simulink model "Planta_5_8_24"  (R2021a)
settings: Solver=VariableStepAuto  StartTime=0.0  StopTime=130  FixedStep=0.002  MaxStep=1e-3  RelTol=1e-4
model workspace (MAT data in the model file):
  VelMin = 0.5
  vMax = -0.3
values from neighbouring files (symbols this model uses):
  ax_max = 0.8    [valoresPlanta_29_9_24.m]    (also in valoresPlanta_v4.m)
  ay_max = 0.75    [valoresPlanta_29_9_24.m]    (also in valoresPlanta_v4.m)
  bcy = 1e7    (= 10000000)    [Valores_1.m]    (also in valoresPlanta.m; valoresPlanta_29_9_24.m; valoresPlanta_V3.m; valoresPlanta_v4.m)
  bh_eq = bhm*ih^2+bhd    (= 8720)    [Valores.m]    (also in Valores_1.m; valoresPlanta.m; valoresPlanta_29_9_24.m; valoresPlanta_V3.m)
  bhb = 1e8    (= 100000000)    [Valores.m]    (also in Valores_1.m; valoresPlanta.m; valoresPlanta_29_9_24.m; valoresPlanta_V3.m)
  bhEb = 2.2e9    (= 2200000000)    [Valores.m]    (also in Valores_1.m; valoresPlanta.m; valoresPlanta_29_9_24.m; valoresPlanta_V3.m)
  bt = 90.0    (= 90)    [Valores.m]    (also in Valores_1.m; valoresPlanta.m; valoresPlanta_29_9_24.m; valoresPlanta_V3.m)
  bt_eq = btd+(btm*(it^2))    (= 5401.8)    [valoresPlanta.m]    (also in valoresPlanta_29_9_24.m; valoresPlanta_V3.m; valoresPlanta_v4.m)
  btb = 5e6    (= 5000000)    [Valores.m]    (also in Valores_1.m; valoresPlanta.m; valoresPlanta_29_9_24.m; valoresPlanta_V3.m)
  btw = 3.0e3    (= 3000)    [Valores.m]    (also in Valores_1.m; valoresPlanta.m; valoresPlanta_29_9_24.m; valoresPlanta_V3.m)
  bwu = 150    [Valores.m]    (also in Valores_1.m; valoresPlanta.m; valoresPlanta_29_9_24.m; valoresPlanta_V3.m)
  estado_cont = [x_positions; hy_cont]    [perfilObsaculos.m]    (also in valoresPlanta_29_9_24.m = [x_positions; [hy_muelle hy_cont]]; valoresPlanta_v4.m = [x_positions; [hy_muelle hy_cont]])
  g = 9.80665    [Valores.m]    (also in Valores_1.m; valoresPlanta.m; valoresPlanta_29_9_24.m; valoresPlanta_V3.m)
  Hc = 0    [Valores.m]    (also in Valores_1.m = 2.5; valoresPlanta.m = 2.5; valoresPlanta_29_9_24.m = 2.5; valoresPlanta_V3.m = 2.5)
  hx_cont = 2.5    [perfilObsaculos.m]    (also in puntosTrayectoria.m; valoresPlanta_29_9_24.m; valoresPlanta_v4.m)
  ih = 22    [Valores.m]    (also in Valores_1.m; valoresPlanta.m; valoresPlanta_29_9_24.m; valoresPlanta_V3.m)
  it = 30    [Valores.m]    (also in Valores_1.m; valoresPlanta.m; valoresPlanta_29_9_24.m; valoresPlanta_V3.m)
  Jh_eq = Jhm_hb*ih^2+Jhd_hEb    (= 18320)    [Valores.m]    (also in Valores_1.m; valoresPlanta.m; valoresPlanta_29_9_24.m; valoresPlanta_V3.m)
  Jt_eq = Jtd+(Jtm_tb*(it^2))    (= 7500)    [valoresPlanta.m]    (also in valoresPlanta_29_9_24.m; valoresPlanta_V3.m; valoresPlanta_v4.m)
  kcy = 1.8e9    (= 1800000000)    [Valores_1.m]    (also in valoresPlanta.m; valoresPlanta_29_9_24.m; valoresPlanta_V3.m; valoresPlanta_v4.m)
  KDh = Jeq2 * w_posh^3    (= -12245.4404091)    [Valores.m]    (also in Valores_1.m = Jeq2 * w_posh; valoresPlanta.m = Jeq2 * w_posh; valoresPlanta_29_9_24.m = Jh_eq * n * w_posh; valoresPlanta_V3.m = Jeq2 * w_posh)
  KDt = Meq2 * w_post^3    (= -4728.86946035)    [Valores.m]    (also in Valores_1.m = Meq2 * w_post; valoresPlanta.m = Meq2 * w_post; valoresPlanta_29_9_24.m = 10127; valoresPlanta_V3.m = Meq2 * w_post)
  KIh = Jeq2 * w_posh^2    (= 2572.66592082)    [Valores.m]    (also in Valores_1.m = Jeq2 * w_posh^3; valoresPlanta.m = Jeq2 * w_posh^3; valoresPlanta_29_9_24.m = Jh_eq * w_posh^3; valoresPlanta_V3.m = Jeq2 * w_posh^3)
  KIt = Meq2 * w_post^2    (= 1307.690244)    [Valores.m]    (also in Valores_1.m = Meq2 * w_post^3; valoresPlanta.m = Meq2 * w_post^3; valoresPlanta_29_9_24.m = 6809.6; valoresPlanta_V3.m = Meq2 * w_post^3)
  KPh = Jeq2 * w_posh    (= -540.495867769)    [Valores.m]    (also in Valores_1.m = Jeq2 * w_posh^2; valoresPlanta.m = Jeq2 * w_posh^2; valoresPlanta_29_9_24.m = Jh_eq * n * w_posh^2; valoresPlanta_V3.m = Jeq2 * w_posh^2)
  KPt = Meq2 * w_post    (= -361.62)    [Valores.m]    (also in Valores_1.m = Meq2 * w_post^2; valoresPlanta.m = Meq2 * w_post^2; valoresPlanta_29_9_24.m = 14123; valoresPlanta_V3.m = Meq2 * w_post^2)
  Ktw = 4.8e5    (= 480000)    [Valores.m]    (also in Valores_1.m; valoresPlanta.m; valoresPlanta_29_9_24.m; valoresPlanta_V3.m)
  kwu = 2.36e8    (= 236000000)    [Valores.m]    (also in Valores_1.m; valoresPlanta.m; valoresPlanta_29_9_24.m; valoresPlanta_V3.m)
  Mc_max = 5e4    (= 50000)    [Valores.m]    (also in Valores_1.m; valoresPlanta.m; valoresPlanta_29_9_24.m; valoresPlanta_V3.m)
  Mc_min = 2e3    (= 2000)    [Valores.m]    (also in Valores_1.m; valoresPlanta.m; valoresPlanta_29_9_24.m; valoresPlanta_V3.m)
  Meq = Mt+(it^2*Jtm_tb+Jtd)/rtd^2    (= 60000)    [Valores.m]    (also in Valores_1.m; valoresPlanta_29_9_24.m; valoresPlanta_v4.m)
  Ms = 1.5e4    (= 15000)    [Valores.m]    (also in Valores_1.m; valoresPlanta.m; valoresPlanta_29_9_24.m; valoresPlanta_V3.m)
  Mt = 30000    [Valores.m]    (also in Valores_1.m; valoresPlanta.m; valoresPlanta_29_9_24.m; valoresPlanta_V3.m)
  pos = [p0; p1; p2; p3; p4; p5]    [calcularTrayectoria2_prueba.m]    (also in perfilObsaculos.m = puntosTrayectoria(4, 1.5, 20, [-20,0], estado_cont, hy_cont,; puntosTrayectoria.m; valoresPlanta_29_9_24.m = calcularTrayectoria2_prueba(vx_max, vhmax, ax_max, Hc, hx_co; valoresPlanta_v4.m = calcularTrayectoria2_prueba(vx_max, vhmax, ax_max, Hc, hx_co)
  rhd = 0.75    [Valores.m]    (also in Valores_1.m; valoresPlanta.m; valoresPlanta_29_9_24.m; valoresPlanta_V3.m)
  rtd = 0.5    [Valores.m]    (also in Valores_1.m; valoresPlanta.m; valoresPlanta_29_9_24.m; valoresPlanta_V3.m)
  tau_hm = 1e-3    (= 0.001)    [valoresPlanta.m]    (also in valoresPlanta_29_9_24.m; valoresPlanta_V3.m; valoresPlanta_v4.m)
  tau_tm = 1e-3    (= 0.001)    [Valores.m]    (also in Valores_1.m; valoresPlanta.m; valoresPlanta_29_9_24.m; valoresPlanta_V3.m)
  Thb_Max = 5e4    (= 50000)    [Valores.m]    (also in Valores_1.m; valoresPlanta.m; valoresPlanta_29_9_24.m; valoresPlanta_V3.m)
  ThEb_Max = 1.1e6    (= 1100000)    [Valores.m]    (also in Valores_1.m; valoresPlanta.m; valoresPlanta_29_9_24.m; valoresPlanta_V3.m)
  Thm_Max = 2e4    (= 20000)    [Valores.m]    (also in Valores_1.m; valoresPlanta.m; valoresPlanta_29_9_24.m; valoresPlanta_V3.m)
  Ttb_Max = 5e3    (= 5000)    [Valores.m]    (also in Valores_1.m; valoresPlanta.m; valoresPlanta_29_9_24.m; valoresPlanta_V3.m)
  Ttm_Max = 3e3    (= 3000)    [Valores.m]    (also in Valores_1.m; valoresPlanta.m; valoresPlanta_29_9_24.m = 4000; valoresPlanta_V3.m)
  vhmax = 3    [valoresPlanta_29_9_24.m]    (also in valoresPlanta_V3.m; valoresPlanta_v4.m)
  vx_max = 4    [valoresPlanta_29_9_24.m]    (also in valoresPlanta_v4.m)
  whmMax = P/Thm_Max    (= 47.8075)    [Valores_1.m]    (also in valoresPlanta.m; valoresPlanta_29_9_24.m = 176; valoresPlanta_V3.m; valoresPlanta_v4.m = 176)
  whmMin = 0.02    [valoresPlanta_29_9_24.m]    (also in valoresPlanta_v4.m = 0.2)
  wtmMax = (4/rtd)*it    (= 240)    [Valores_1.m]    (also in valoresPlanta.m; valoresPlanta_29_9_24.m; valoresPlanta_V3.m; valoresPlanta_v4.m)
  wtmMin = 0.02    [valoresPlanta_29_9_24.m]    (also in valoresPlanta_v4.m = 0.2)
  x_0 = -20    [valoresPlanta_29_9_24.m]    (also in valoresPlanta_v4.m)
  x_0_tamb = x_0/rtd    (= -40)    [valoresPlanta_29_9_24.m]    (also in valoresPlanta_v4.m)
  xLimMax = 49    [valoresPlanta_29_9_24.m]    (also in valoresPlanta_v4.m)
  xLimMaxSeguridad = 50    [valoresPlanta_29_9_24.m]    (also in valoresPlanta_v4.m)
  xLimMin = -29    [valoresPlanta_29_9_24.m]    (also in valoresPlanta_v4.m)
  xLimMinSeguridad = -30    [valoresPlanta_29_9_24.m]    (also in valoresPlanta_v4.m)
  y_0 = 2.5    [valoresPlanta_29_9_24.m]    (also in valoresPlanta_v4.m)
  y_0_izaje = 3*(2/rhd)    (= 8)    [valoresPlanta_29_9_24.m]    (also in valoresPlanta_v4.m)
  yLimMax = 44    [valoresPlanta_29_9_24.m]    (also in valoresPlanta_v4.m)
  yLimMaxSeguridad = 45    [valoresPlanta_29_9_24.m]    (also in valoresPlanta_v4.m)
  yLimMin = -19    [valoresPlanta_29_9_24.m]    (also in valoresPlanta_v4.m)
  yLimMinSeguridad = -20    [valoresPlanta_29_9_24.m]    (also in valoresPlanta_v4.m)
  Yt0 = 45    [Valores.m]    (also in Valores_1.m; valoresPlanta.m; valoresPlanta_29_9_24.m; valoresPlanta_V3.m)
undefined symbols (not defined in the file or in its folder): DiscIntNeverNeededParam
libraries: simulink x3, vrlib x1, simulink_extras x1, aerolibanimutils x1
(part 2 of 3)

== system Planta_5_8_24/Planta/Modulador de Torque ==
  note: Modulador de Torque
  Ttm_ : Inport
  whd : Inport  Port=2
  wtd : Inport  Port=3
  T_hm_0 : Inport  Port=4
  Thm_ : Inport  Port=5
  Gain : Gain  Gain=bh_eq
  Gain1 : Gain  Gain=bt_eq
  Modulador de Torque Carro : Subsystem
  Modulador de Torque Izaje : Subsystem
  Saturation6 : Saturate  UpperLimit=Ttm_Max  LowerLimit=-Ttm_Max
  Saturation7 : Saturate  UpperLimit=Thm_Max  LowerLimit=-Thm_Max
  Scope29 : Scope
  Sum : Sum  Inputs=|++
  Sum3 : Sum  Inputs=|++
  Ttm(t) : Outport
  Thm(t) : Outport  Port=2
  wires:
  T_hm_0/1 -> Modulador de Torque Izaje/1(T_hm_0)
  Gain/1 -> Sum/2
  Sum/1 -> Saturation7/1
  wtd/1 -> Gain1/1
  Saturation6/1 -> Modulador de Torque Carro/1(Ttm*(t))
  Saturation7/1 -> Modulador de Torque Izaje/2(Thm*(t))
  Sum3/1 -> Scope29/1, Saturation6/1
  Gain1/1 -> Sum3/2
  Ttm_/1 -> Sum3/1
  Modulador de Torque Izaje/1(Thm(t)) -> Thm(t)/1
  whd/1 -> Gain/1
  Modulador de Torque Carro/1(Ttm(t)) -> Ttm(t)/1
  Thm_/1 -> Sum/1

== system Planta_5_8_24/Planta/Subsistema Carro ==
  theta(t) : Inport
  Fhw(t) : Inport  Port=2
  Ftw(t) : Inport  Port=3
  Constant : Constant  Value=x_0
  Gain : Gain  Gain=1/Mt
  Gain1 : Gain  Gain=2
  Gain2 : Gain  Gain=bt
  Integrator : Integrator
  Integrator1 : Integrator  InitialConditionSource=external
  Product : Product
  Sin : Trigonometry
  Sum : Sum  Inputs=++-
  xt(t) : Outport
  vt(t) : Outport  Port=2
  at(t) : Outport  Port=3
  wires:
  Integrator/1 -> vt(t)/1, Integrator1/1, Gain2/1
  Gain1/1 -> Product/2
  theta(t)/1 -> Sin/1
  Sum/1 -> Gain/1
  Product/1 -> Sum/1
  Integrator1/1 -> xt(t)/1
  Ftw(t)/1 -> Sum/2
  Gain2/1 -> Sum/3
  Fhw(t)/1 -> Gain1/1
  Sin/1 -> Product/1
  Constant/1 -> Integrator1/2
  Gain/1 -> at(t)/1, Integrator/1

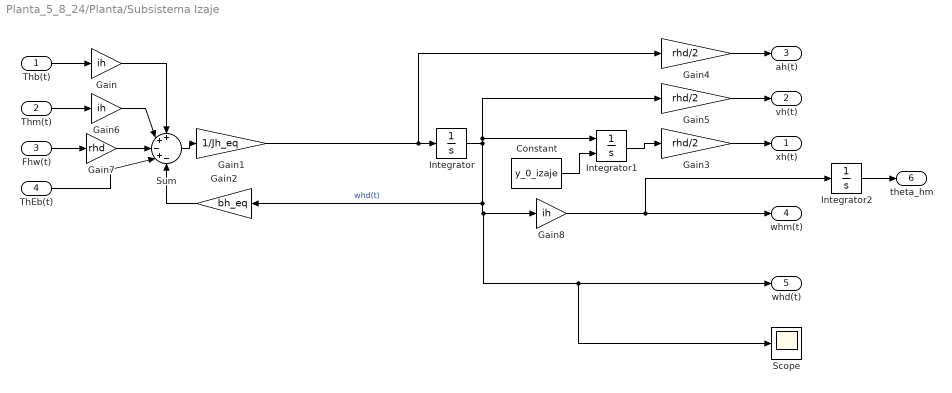
== system Planta_5_8_24/Planta/Subsistema Izaje ==
  Thb(t) : Inport
  Thm(t) : Inport  Port=2
  Fhw(t) : Inport  Port=3
  ThEb(t) : Inport  Port=4
  Constant : Constant  Value=y_0_izaje
  Gain : Gain  Gain=ih
  Gain1 : Gain  Gain=1/Jh_eq
  Gain2 : Gain  Gain=bh_eq
  Gain3 : Gain  Gain=rhd/2
  Gain4 : Gain  Gain=rhd/2
  Gain5 : Gain  Gain=rhd/2
  Gain6 : Gain  Gain=ih
  Gain7 : Gain  Gain=rhd
  Gain8 : Gain  Gain=ih
  Integrator : Integrator
  Integrator1 : Integrator  InitialConditionSource=external
  Integrator2 : Integrator
  Scope : Scope
  Sum : Sum  Inputs=++-+-
  xh(t) : Outport
  vh(t) : Outport  Port=2
  ah(t) : Outport  Port=3
  whm(t) : Outport  Port=4
  whd(t) : Outport  Port=5
  theta_hm : Outport  Port=6
  wires:
  Integrator/1 -> Gain5/1, Integrator1/1, Scope/1, whd(t)/1, Gain8/1, Gain2/1  "whd(t)"
  Gain2/1 -> Sum/5
  Gain4/1 -> ah(t)/1
  Gain3/1 -> xh(t)/1
  Gain5/1 -> vh(t)/1
  Fhw(t)/1 -> Gain7/1
  Integrator1/1 -> Gain3/1
  Thb(t)/1 -> Gain/1
  Sum/1 -> Gain1/1
  Thm(t)/1 -> Gain6/1
  Gain/1 -> Sum/1
  Gain6/1 -> Sum/2
  Gain7/1 -> Sum/3
  ThEb(t)/1 -> Sum/4
  Gain8/1 -> Integrator2/1, whm(t)/1
  Constant/1 -> Integrator1/2
  Gain1/1 -> Gain4/1, Integrator/1
  Integrator2/1 -> theta_hm/1

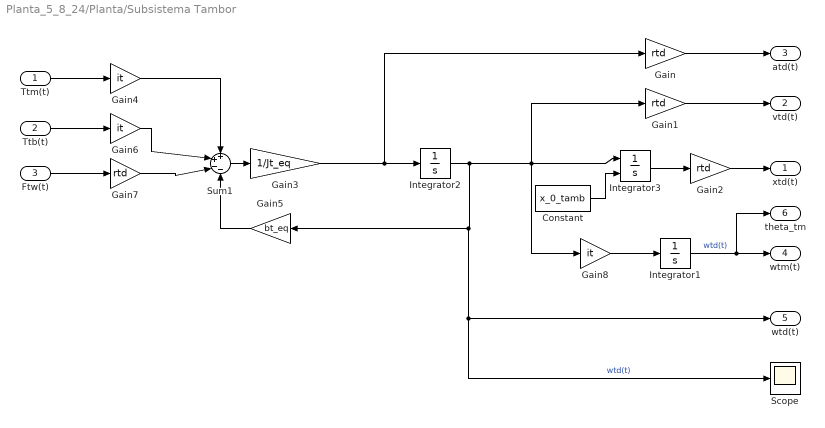
== system Planta_5_8_24/Planta/Subsistema Tambor ==
  Ttm(t) : Inport
  Ttb(t) : Inport  Port=2
  Ftw(t) : Inport  Port=3
  Constant : Constant  Value=x_0_tamb
  Gain{,1..2,7} (4 alike) : Gain  Gain=rtd
  Gain3 : Gain  Gain=1/Jt_eq
  Gain4 : Gain  Gain=it
  Gain5 : Gain  Gain=bt_eq
  Gain6 : Gain  Gain=it
  Gain8 : Gain  Gain=it
  Integrator1 : Integrator
  Integrator2 : Integrator
  Integrator3 : Integrator  InitialConditionSource=external
  Scope : Scope
  Sum1 : Sum  Inputs=++--
  xtd(t) : Outport
  vtd(t) : Outport  Port=2
  atd(t) : Outport  Port=3
  wtm(t) : Outport  Port=4
  wtd(t) : Outport  Port=5
  theta_tm : Outport  Port=6
  wires:
  Integrator3/1 -> Gain2/1
  Ftw(t)/1 -> Gain7/1
  Gain2/1 -> xtd(t)/1
  Integrator2/1 -> Gain1/1, Integrator3/1, Gain8/1, Scope/1, wtd(t)/1, Gain5/1  "wtd(t)"
  Ttm(t)/1 -> Gain4/1
  Ttb(t)/1 -> Gain6/1
  Sum1/1 -> Gain3/1
  Gain5/1 -> Sum1/4
  Gain1/1 -> vtd(t)/1
  Gain/1 -> atd(t)/1
  Gain4/1 -> Sum1/1
  Gain6/1 -> Sum1/2
  Gain7/1 -> Sum1/3
  Gain8/1 -> Integrator1/1
  Constant/1 -> Integrator3/2
  Gain3/1 -> Integrator2/1, Gain/1
  Integrator1/1 -> theta_tm/1, wtm(t)/1  "wtd(t)"

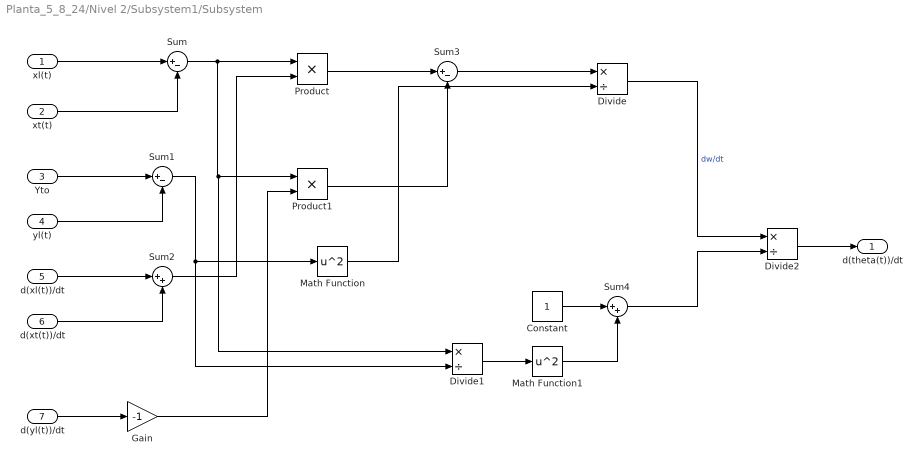
== system Planta_5_8_24/Nivel 2/Subsystem1/Subsystem ==
  xl(t) : Inport
  xt(t) : Inport  Port=2
  Yto : Inport  Port=3
  yl(t) : Inport  Port=4
  d(xl(t))/dt : Inport  Port=5
  d(xt(t))/dt : Inport  Port=6
  d(yl(t))/dt : Inport  Port=7
  Constant : Constant
  Divide : Product  Inputs=*/
  Divide1 : Product  Inputs=*/
  Divide2 : Product  Inputs=*/
  Gain : Gain  Gain=-1
  Math Function : Math  Operator=square  SaturateOnIntegerOverflow=on
  Math Function1 : Math  Operator=square  SaturateOnIntegerOverflow=on
  Product : Product
  Product1 : Product
  Sum : Sum  Inputs=|+-
  Sum1 : Sum  Inputs=|+-
  Sum2 : Sum  Inputs=|++
  Sum3 : Sum  Inputs=|+-
  Sum4 : Sum  Inputs=|++
  d(theta(t))/dt : Outport
  wires:
  xl(t)/1 -> Sum/1
  xt(t)/1 -> Sum/2
  Yto/1 -> Sum1/1
  yl(t)/1 -> Sum1/2
  Sum/1 -> Divide1/1, Product1/1, Product/1
  d(xl(t))/dt/1 -> Sum2/1
  d(xt(t))/dt/1 -> Sum2/2
  Sum2/1 -> Product/2
  Product/1 -> Sum3/1
  Product1/1 -> Sum3/2
  d(yl(t))/dt/1 -> Gain/1
  Gain/1 -> Product1/2
  Sum3/1 -> Divide/1
  Sum1/1 -> Math Function/1, Divide1/2
  Math Function/1 -> Divide/2
  Divide/1 -> Divide2/1  "dw/dt"
  Divide1/1 -> Math Function1/1
  Math Function1/1 -> Sum4/2
  Constant/1 -> Sum4/1
  Divide2/1 -> d(theta(t))/dt/1
  Sum4/1 -> Divide2/2

== system Planta_5_8_24/Planta/Modulador de Torque/Modulador de Torque Carro ==
  Ttm*(t) : Inport
  Gain1 : Gain  Gain=1/tau_tm
  Integrator : Integrator
  Sum : Sum  Inputs=|+-
  Ttm(t) : Outport
  wires:
  Gain1/1 -> Integrator/1
  Integrator/1 -> Ttm(t)/1, Sum/2
  Ttm*(t)/1 -> Sum/1
  Sum/1 -> Gain1/1

== system Planta_5_8_24/Planta/Modulador de Torque/Modulador de Torque Izaje ==
  T_hm_0 : Inport
  Thm*(t) : Inport  Port=2
  Gain1 : Gain  Gain=1/tau_hm
  Integrator : Integrator  InitialConditionSource=external
  Sum : Sum  Inputs=|+-
  Thm(t) : Outport
  wires:
  Gain1/1 -> Integrator/1
  Integrator/1 -> Thm(t)/1, Sum/2
  Thm*(t)/1 -> Sum/1
  Sum/1 -> Gain1/1
  T_hm_0/1 -> Integrator/2

== stateflow chart Planta_5_8_24/Chart ==
  state AUTOMATICO
    entry:
    automatic=1;
  state MANUAL
    entry:
    automatic=0;
  (default) -> MANUAL
  AUTOMATICO -> MANUAL : [RB==1 ]
  MANUAL -> AUTOMATICO : [RB==1]
  data: automatic output; RB input

== matlab function Planta_5_8_24/Planta/MATLAB Function ==
  data: index output; estado_cont input; y_evol output; xl input; anchoCont input
function [index, y_evol] = envolvente(estado_cont, xl, anchoCont)
%Calculo de envolvente. Hay un perfil de contenedores. 
%Se debe usar la posicion actual de la carga para comparar con la altura
%que debe tener el contenedor (teniendo en cuenta el indice del vector)
%si la carga esta entre los limites del contenedor(i) (contenedor(i) -
%contenedor(i)aX*0.5 y contenedor(i) + contenedor(i)aX*0.5)
% Dividir la posicion en x de la carga por el ancho de contenedores para
% obtener la posicion del indice  (usar floor?) --> si da 0 por ejemplo la
% la altura del envolvente sera igual a la del contenedor en el indice 0
% mas el factor de seguridad. Para el modo de contacto no usar el factor de
% seguridad.
fseg = 0;  %2.5;  Buscar si no esta guardado previamente
index = floor((xl)/anchoCont)+13;   %revisar +1
%si xl es menor a 0 (con las posiciones corregidas, sin el offset,
%modificar los valores para que sean 0 (muelle) o la altura de un camion

%% index: puedo hacer que compare index con index anterior
    if (index<=0)
        y_evol = 0; %-6+fseg; %por ahora solo muelle, si uso 0 entra directo en modo contancto

    elseif (index>0 && index<32)
    %     y_evol = con(index) + fseg;
        y_evol = estado_cont(2,index) + fseg;
    elseif (index>32)
        %no deberia pasar 
        y_evol = -5+fseg;
    else
        y_evol = 0;
    end




end

== stateflow chart Planta_5_8_24/graficos ==
  state Graficar
    entry:
    cont = 0;
    %contenedor = rectangle('Position',[xl-2.25, yl, 4.5, 2.5 ],'FaceColor','g');
    %carro = rectangle('Position',[xt-2, Yt0, 4.5, 2 ],'FaceColor','r');
    during:
    dock_shore_graph(xt, xl, yl, Yt0,Hc,cont);
    cont = cont+1;
  (default) -> Graficar
  data: Xt function_input; Xl function_input; Yl function_input; YT0 function_input; HC function_input; Con function_input; Hc input; Yt0 input; xl input; xt input; yl input; cont local
  function dock_shore_graph(Xt, Xl, Yl, YT0, HC,Con):
    | function dock_shore_graph(Xt, Xl, Yl, YT0, HC,Con)
    | %viga voladiza
    | plot([-30 50],[45 45 ],'Color','k')
    | hold on
    | %cable
    | cable = plot([xt xl],[45 yl+Hc],'Color','k');
    | %carro (modificar luego)
    | carro = rectangle('Position',[xt-2, Yt0, 4.5, 2 ],'FaceColor','r');
    | %Conenedor
    | contenedor = rectangle('Position',[xl-2.25, yl, 4.5, 2.5 ],'FaceColor','g');
    | %barco
    | rectangle('Position',[2, -20.5, 0.5, 25.5 ],'FaceColor','b');
    | rectangle('Position',[50, -20.5, 0.5, 25.5 ],'FaceColor','b');
    | rectangle('Position',[2, -20.5, 48, 0.5 ],'FaceColor','b');
    | %muelle
    | rectangle('Position',[-30, -0.5, 30, 0.5 ],'FaceColor','k');
    | rectangle('Position',[0, -20, 0.5, 20 ],'FaceColor','k');
    | 
    | title("Operacion de carga y descarga");
    | xlabel("Distancia (mts)");
    | ylabel("Altura (mts)");
    | hold on
    | if (cont>0)
    |     set(carro, 'Position', [xt-2, Yt0, 4.5, 2 ]);
    |     set(contenedor, 'Position', [xl-2.25, yl, 4.5, 2.5 ]);
    |     set(cable,'XData', [xt xl], 'YData', [45 yl]);
    |     %cable = plot([xt xl],[45 yl],'Color','k');
    | end
    | % %perfil de contenedores VARIABLE
    | % x = 6.5:5:46.5;
    | % y = [15 20 32 16 35 11 32 22 10];
    | % b = bar(x,y); %,'histc'
    | % b(1).BaseValue = -20;
    | % b(1).BaseLine.LineWidth = 0.01;
    | % b(1).ShowBaseLine=0;
    | % b(1).BarWidth=0.9;
    | % b(1).FaceColor = [0.8500 0.3250 0.0980];
    | % % Actualizar los datos del gráfico de barras
    | % set(b, 'YData', datos);
    | %---------------------------------------------------
    | % Perfil de contenedores
    | puntos_iniciales = [5 -20; 10 -20; 15 -20; 20 -20; 25 -20; 30 -20; 35 -20; 40 -20; 45 -20];
    | % Definir las dimensiones de los rectángulos
    | dimensiones = [15; 12; 20; 18; 14; 16; 13; 10; 8];
    | 
    | % Bucle para crear los rectángulos
    | for i = 1:size(puntos_iniciales, 1)
    |     % Obtener las coordenadas del punto inicial
    |     x = puntos_iniciales(i, 1);
    |     y = puntos_iniciales(i, 2);
    |     altura = dimensiones(i);
    |     % Crear el rectángulo utilizando el comando 'rectangle'
    |     rectangle('Position', [x, y, 5, altura], 'FaceColor', 'red');
    |     
    | %     hold on; % Para mantener los rectángulos en el gráfico
    | end
    | 
    | % Refrescar el gráfico
    | drawnow;
    | 
    | % Pausa para observar el cambio en el gráfico
    | pause(0.5);
    | set(carro, 'visible', 'off');
    | set(contenedor, 'visible', 'off');
    | set(cable, 'visible', 'off');
    | % if (mod(cont,7)==0)
    | %     set(carro, 'visible', 'off');
    | %     set(contenedor, 'visible', 'off');
    | %     %carro (modificar luego)
    | % carro = rectangle('Position',[xt-2, Yt0, 4.5, 2 ],'FaceColor','r');
    | % %Conenedor
    | % contenedor = rectangle('Position',[xl-2.25, yl, 4.5, 2.5 ],'FaceColor','g');
    | % end
    | end

== stateflow chart Planta_5_8_24/Nivel 0 ==
  state Nivel_0
    entry:
    alerta = 0;
    state WATCHDOG [parallel]
      settings: executionOrder=2
      state RESET_TIMER
        entry:
        wd_timer=0;
        alerta=0;
      state Flanco_subida
        during:
        wd_timer = wd_timer + 1;
      state Flanco_Bajada
        during:
        wd_timer = wd_timer + 1;
      state Estado_Emergencia
        entry:
        alerta=1;
        Emergencia = 1;
      (default) -> RESET_TIMER
      Estado_Emergencia -> RESET_TIMER : [RESET == 1]
      Flanco_Bajada -> RESET_TIMER [order 2] : [~wd_signal]
      RESET_TIMER -> Flanco_subida : [~wd_signal]
      Flanco_subida -> Flanco_Bajada [order 2] : [wd_signal]
      Flanco_subida -> Estado_Emergencia [order 1] : [wd_timer>WD_TIMEOUT]
      Flanco_Bajada -> Estado_Emergencia [order 1] : [wd_timer>WD_TIMEOUT]
    state Control [parallel]
      settings: executionOrder=1
      state EmergenciaCarro
        entry:
        pBRKh = 1;
        pBRKt = 0;
        pBRKEh = 1;
        Balanceo = 0;
        Emergencia =1;
      state EstadoNormal
        entry:
        pBRKh = 1;
        pBRKt = 1;
        pBRKEh = 1;
        Balanceo = 1;
        Emergencia = 0;
      state EmergenciaGlobal
        during:
        %1 porque es pulsador. no freno
        pBRKh = 0;
        pBRKt = 0;
        pBRKEh = 0;
        Balanceo = 0;
        Emergencia =1;
      state EmergenciaIzaje
        entry:
        pBRKh = 0;
        pBRKt = 1;
        pBRKEh = 1;
        Emergencia = 1;
      (default) -> EstadoNormal
      EstadoNormal -> EmergenciaCarro [order 2] : [(flagFDCtLimInf==1) || (flagFDCtLimSup==1) || (sobrevel_t ==1)]
      EmergenciaCarro -> EstadoNormal [order 1] : [RESET == 1]
      EmergenciaIzaje -> EstadoNormal : [RESET == 1]
      EstadoNormal -> EmergenciaIzaje [order 3] : [(flagFDChLimInf==1) || (flagFDChLimSup==1) || (sobrevel_h==1) || (sobrecarga ==1)]
      EmergenciaGlobal -> EstadoNormal : [pulsadorEmergencia == 0 || alerta ==0]
      EmergenciaCarro -> EmergenciaGlobal [order 2] : [(flagFDChLimInf==1) || (flagFDChLimSup==1) || (sobrevel_h==1)]
      EstadoNormal -> EmergenciaGlobal [order 1] : [pulsadorEmergencia == 1 || alerta ==1]
  data: pulsadorEmergencia input; pBRKEh output; pBRKh output; pBRKt output; Balanceo output; RESET input; Emergencia output double size=1; sobrevel_h input; sobrevel_t input; sobrecarga input; WD_TIMEOUT parameter; wd_signal input; wd_timer local; alerta local; flagFDChLimInf input; flagFDChLimSup input; flagFDCtLimInf input; flagFDCtLimSup input

== stateflow chart Planta_5_8_24/Chart4 ==
  state TWISLOCK_ON
    entry:
    TWIS=1;
  state TWISLOCK_OFF
    entry:
    TWIS=0;
  (default) -> TWISLOCK_OFF
  TWISLOCK_ON -> TWISLOCK_OFF : [LB==1 ]
  TWISLOCK_OFF -> TWISLOCK_ON : [LB==1]
  data: TWIS output; LB input

== stateflow chart Planta_5_8_24/Planta/Modo Twistlocks ==
  state TLK_OFF
    entry:
    hc=0;
    ml=Ms;
  state TLK_ON
    entry:
    hc=2.5;
    ml=Ms+Mcx;
  (default) -> TLK_OFF
  TLK_OFF -> TLK_ON : [tw == 1]
  TLK_ON -> TLK_OFF : [tw==0]
  data: Mcx input; hc output; Ms parameter; ml output; tw input
